simulink model "simulation_Nonlinear_ship_moving_target_ALL"  (R2024b)
settings: Solver=VariableStepAuto  StartTime=0.0  StopTime=30  RelTol=1e-3
libraries: simulink x3
settings Model: Creator=Omer Mizrachi  LastModifiedBy=alonorlicky

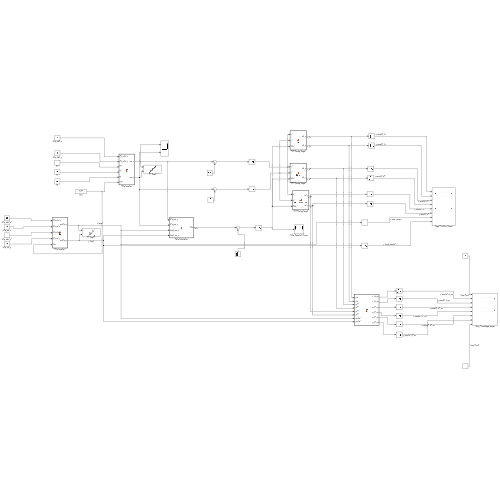
[thumbnail: Simulink's stored preview of the top-level diagram]
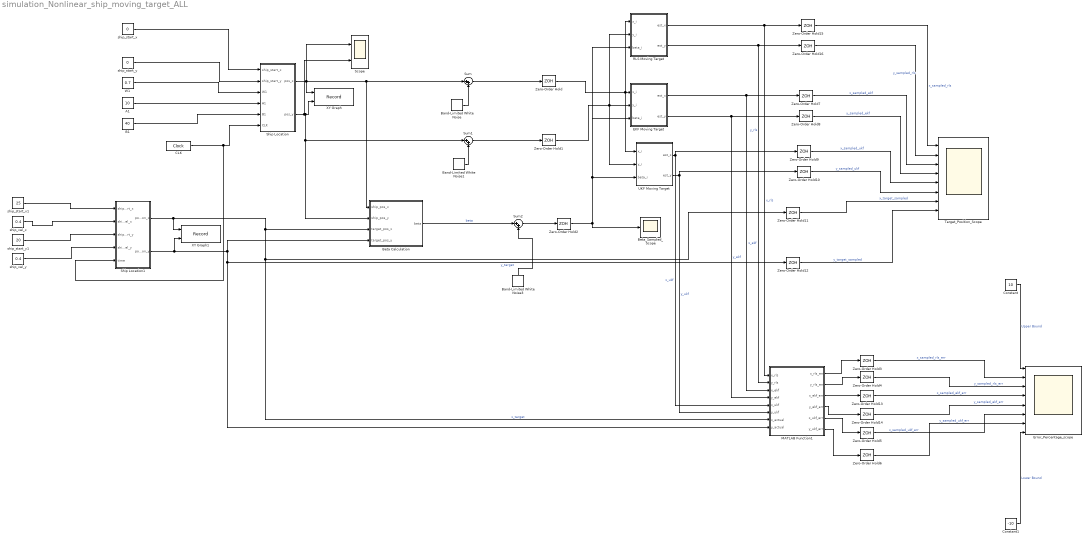
== system simulation_Nonlinear_ship_moving_target_ALL ==
  A1 : Constant  Value=10
  B1 : Constant  Value=40
  Band-Limited White Noise : simulink/Sources/Band-Limited White Noise  Cov=[1.2]  Ts=0.01  seed=[23341]
  Band-Limited White Noise1 : simulink/Sources/Band-Limited White Noise  Cov=[1.2]  Ts=0.01  seed=[233471]
  Band-Limited White Noise3 : simulink/Sources/Band-Limited White Noise  Cov=[ 0.0001]  Ts=0.01  seed=[21113341]
  Beta Calculation : MATLAB Function  TreatAsAtomicUnit=on
  Beta_Sampled_Scope : Scope
  CLK : DigitalClock  SampleTime=0.01
  Constant : Constant  Value=10
  Constant1 : Constant  Value=-10
  EKF Moving Target : MATLAB Function  TreatAsAtomicUnit=on
  Error_Percentage_scope : Scope  NumInputPorts=8
  MATLAB Function1 : MATLAB Function  TreatAsAtomicUnit=on
  RLS Moving Target : MATLAB Function  TreatAsAtomicUnit=on
  Scope : Scope  NumInputPorts=2
  Ship Location : MATLAB Function  TreatAsAtomicUnit=on
  Ship Location1 : MATLAB Function  TreatAsAtomicUnit=on
  Sum : Sum  Inputs=|++
  Sum1 : Sum  Inputs=|++
  Sum2 : Sum  Inputs=|++
  Target_Position_Scope : Scope  NumInputPorts=8
  UKF Moving Target : MATLAB Function  TreatAsAtomicUnit=on
  W1 : Constant  Value=0.7
  XY Graph : Record  FileSettingsInternal="{\"entries\":[{\"content\":{\"excelSettings\":{\"content\":{},\"type\":\"Streamout.ExcelSettings\"}},\"type\":\"Streamout.FileSettingStorage\",\"uuid\":\"\"}],\"packageUris\":[\"http:\\/\\/schema.mathworks.com\\/mf0\\/streamout_blocks\\/R2020a\"],\"version\":\"1.0\"}"  Layout=[1 1]  SignalsInternal="{\"entries\":[{\"content\":{\"signals\":[{\"content\":{\"blockPath\":[],\"dimensions\":[1],\"domain\":\"\",\"lineColor\":\"#0072bd\",\"lineWidth\":2,\"plots\":[ 1 ],\"port\":1,\"sid\":[\"\"],\"signalID\":1,\"signalName\":\"Ship Location:1\"},\"type\":\"RecordBlkView.Signal\",\"uuid\":\"\"},{\"content\":{\"blockPath\":[],\"dimensions\":[1],\"domain\":\"\",\"lineColor\":\"#d95319\",\"lineWidth\":2,\"plots\":[ 1 ],\"port\":2,\"sid\":[\"\"],\"signalID\":2,\"signalName\":\"Ship Location:2\"},\"type\":\"RecordBlkView.Signal\",\"uuid\":\"\"}]},\"type\":\"RecordBlkView.InputSignals\",\"uuid\":\"\"}],\"packageUris\":[\"http:\\/\\/schema.mathworks.com\\/mf0\\/streamout_blocks\\/R2020a\"],\"version\":\"1.0\"}"  VisualizationBindings="{\"xyplotplugin\":{\"info\":[{\"series\":[{\"bindingParametersList\":[{\"parameter\":\"X-Axis\",\"signalID\":1,\"signalName\":\"Ship Location:1\"},{\"parameter\":\"Y-Axis\",\"signalID\":2,\"signalName\":\"Ship Location:2\"}],\"seriesID\":0}],\"subplotID\":1}]}}"  CompatibilityTag=XY
  XY Graph1 : Record  FileSettingsInternal="{\"entries\":[{\"content\":{\"excelSettings\":{\"content\":{},\"type\":\"Streamout.ExcelSettings\"}},\"type\":\"Streamout.FileSettingStorage\",\"uuid\":\"\"}],\"packageUris\":[\"http:\\/\\/schema.mathworks.com\\/mf0\\/streamout_blocks\\/R2020a\"],\"version\":\"1.0\"}"  Layout=[1 1]  SignalsInternal="{\"entries\":[{\"content\":{\"signals\":[{\"content\":{\"blockPath\":[],\"dimensions\":[1],\"domain\":\"\",\"lineColor\":\"#0072bd\",\"lineWidth\":2,\"plots\":[ 1 ],\"port\":1,\"sid\":[\"\"],\"signalID\":1,\"signalName\":\"x_target\"},\"type\":\"RecordBlkView.Signal\",\"uuid\":\"\"},{\"content\":{\"blockPath\":[],\"dimensions\":[1],\"domain\":\"\",\"lineColor\":\"#d95319\",\"lineWidth\":2,\"plots\":[ 1 ],\"port\":2,\"sid\":[\"\"],\"signalID\":2,\"signalName\":\"y_target\"},\"type\":\"RecordBlkView.Signal\",\"uuid\":\"\"}]},\"type\":\"RecordBlkView.InputSignals\",\"uuid\":\"\"}],\"packageUris\":[\"http:\\/\\/schema.mathworks.com\\/mf0\\/streamout_blocks\\/R2020a\"],\"version\":\"1.0\"}"  VisualizationBindings="{\"xyplotplugin\":{\"info\":[{\"series\":[{\"bindingParametersList\":[{\"parameter\":\"X-Axis\",\"signalID\":1,\"signalName\":\"x_target\"},{\"parameter\":\"Y-Axis\",\"signalID\":2,\"signalName\":\"y_target\"}],\"seriesID\":0}],\"subplotID\":1}]}}"  CompatibilityTag=XY
  Zero-Order Hold{,1..16} (17 alike) : ZeroOrderHold  SampleTime=0.01
  ship_start_x : Constant  Value=0
  ship_start_x1 : Constant  Value=25
  ship_start_y : Constant  Value=0
  ship_start_y1 : Constant  Value=20
  ship_vel_x : Constant  Value=0.4
  ship_vel_y : Constant  Value=0.4
  wires:
  Ship Location/2(pos_y) -> Scope/2, Sum1/1, Beta Calculation/2(ship_pos_y), XY Graph/2
  Zero-Order Hold14/1 -> Error_Percentage_scope/5  "y_sampled_ekf_err"
  Zero-Order Hold/1 -> RLS Moving Target/1(x_i), UKF Moving Target/1(x_i), EKF Moving Target/1(x_i)
  Band-Limited White Noise1/1 -> Sum1/2
  EKF Moving Target/2(est_y) -> MATLAB Function1/4(y_ekf), Zero-Order Hold8/1  "y_ekf"
  Zero-Order Hold8/1 -> Target_Position_Scope/4  "y_sampled_ekf"
  Ship Location1/2(position_y) -> XY Graph1/2, MATLAB Function1/8(y_actual), Zero-Order Hold12/1, Beta Calculation/4(target_pos_y)  "y_target"
  Sum2/1 -> Zero-Order Hold2/1
  Zero-Order Hold1/1 -> RLS Moving Target/2(y_i), UKF Moving Target/2(y_i), EKF Moving Target/2(y_i)
  Band-Limited White Noise3/1 -> Sum2/2
  Zero-Order Hold11/1 -> Target_Position_Scope/7  "x_target_sampled"
  MATLAB Function1/3(x_ekf_err) -> Zero-Order Hold13/1
  Ship Location/1(pos_x) -> XY Graph/1, Scope/1, Sum/1, Beta Calculation/1(ship_pos_x)
  Sum1/1 -> Zero-Order Hold1/1
  Zero-Order Hold2/1 -> EKF Moving Target/3(beta_i), RLS Moving Target/3(beta_i), UKF Moving Target/3(beta_i), Beta_Sampled_Scope/1
  Sum/1 -> Zero-Order Hold/1
  Zero-Order Hold13/1 -> Error_Percentage_scope/4  "x_sampled_ekf_err"
  Ship Location1/1(position_x) -> XY Graph1/1, Zero-Order Hold11/1, MATLAB Function1/7(x_actual), Beta Calculation/3(target_pos_x)  "x_target"
  Beta Calculation/1(beta) -> Sum2/1  "beta"
  Zero-Order Hold7/1 -> Target_Position_Scope/3  "x_sampled_ekf"
  Zero-Order Hold12/1 -> Target_Position_Scope/8  "y_target_sampled"
  EKF Moving Target/1(est_x) -> MATLAB Function1/3(x_ekf), Zero-Order Hold7/1  "x_ekf"
  MATLAB Function1/4(y_ekf_err) -> Zero-Order Hold14/1
  Band-Limited White Noise/1 -> Sum/2
  Constant1/1 -> Error_Percentage_scope/8  "Lower Bound"
  Constant/1 -> Error_Percentage_scope/1  "Upper Bound"
  UKF Moving Target/2(est_y) -> MATLAB Function1/6(y_ukf), Zero-Order Hold10/1  "y_ukf"
  UKF Moving Target/1(est_x) -> MATLAB Function1/5(x_ukf), Zero-Order Hold9/1  "x_ukf"
  RLS Moving Target/2(est_y) -> MATLAB Function1/2(y_rls), Zero-Order Hold16/1  "y_rls"
  RLS Moving Target/1(est_x) -> Zero-Order Hold15/1, MATLAB Function1/1(x_rls)  "x_rls"
  Zero-Order Hold4/1 -> Error_Percentage_scope/3  "y_sampled_rls_err"
  MATLAB Function1/2(y_rls_err) -> Zero-Order Hold4/1
  MATLAB Function1/1(x_rls_err) -> Zero-Order Hold3/1
  Zero-Order Hold3/1 -> Error_Percentage_scope/2  "x_sampled_rls_err"
  Zero-Order Hold6/1 -> Error_Percentage_scope/7  "y_sampled_ukf_err"
  MATLAB Function1/6(y_ukf_err) -> Zero-Order Hold6/1
  MATLAB Function1/5(x_ukf_err) -> Zero-Order Hold5/1
  Zero-Order Hold5/1 -> Error_Percentage_scope/6  "x_sampled_ukf_err"
  Zero-Order Hold15/1 -> Target_Position_Scope/1  "x_sampled_rls"
  Zero-Order Hold16/1 -> Target_Position_Scope/2  "y_sampled_rls"
  Zero-Order Hold9/1 -> Target_Position_Scope/5  "x_sampled_ukf"
  Zero-Order Hold10/1 -> Target_Position_Scope/6  "y_sampled_ukf"
  B1/1 -> Ship Location/5(B1)
  ship_start_x/1 -> Ship Location/1(ship_start_x)
  W1/1 -> Ship Location/3(W1)
  ship_start_y/1 -> Ship Location/2(ship_start_y)
  A1/1 -> Ship Location/4(A1)
  CLK/1 -> Ship Location1/5(time), Ship Location/6(CLK)
  ship_start_x1/1 -> Ship Location1/1(ship_start_x)
  ship_vel_y/1 -> Ship Location1/4(ship_vel_y)
  ship_vel_x/1 -> Ship Location1/2(ship_vel_x)
  ship_start_y1/1 -> Ship Location1/3(ship_start_y)

== matlab function simulation_Nonlinear_ship_moving_target_ALL/EKF Moving Target ==
  data: x_i input; est_x output; y_i input; beta_i input; est_y output
function [est_x, est_y] = ekf_fcn(x_i, y_i, beta_i)

persistent X_i P Q R


if isempty(P)
    P = 10*eye(8); % Covariance matrix initialization (8x8)
    Q = 0.1*diag([0.001, 0.001, 0.01, 0.001, 0.01, 0.001, 0.01, 0.001]); % Process noise covariance initialization (8x8)
    R = diag([1, 1, 300]); % Measurement noise covariance initialization (3x3)
end
 
if isempty(X_i)
    X_i = zeros(8, 1); % State vector initialization (8x1)
end

dt = 0.01; % Sample time variable
F = [1 dt 0 0 0 0 0 0 ;
     0 1 0 0 0 0 0 0 ; 
     0 0 1 dt 0 0 0 0 ; 
     0 0 0 1 0 0 0 0 ; 
     0 0 0 0 1 dt 0 0 ; 
     0 0 0 0 0 1 0 0 ; 
     0 0 0 0 0 0 1 dt ; 
     0 0 0 0 0 0 0 1]; % Process Jacobian (8x8)
H = [0 0 0 0 1 0 0 0 ; 
    0 0 0 0 0 0 1 0 ; 
    sin(beta_i) 0 -cos(beta_i) 0 -sin(beta_i) 0 cos(beta_i) 0]; % Measurement Jacobian (3x8)

% Prediction Step
X_i = F*X_i; % Process Model
measurement = [x_i ; y_i ; 0]; % Measurements
predicted_measurement = H*X_i; % Measurement Model
P = F*P*F' + Q; % Covariance matrix

% Update Step
innovation = measurement - predicted_measurement; % Measurement residual
K = P*H'/(H*P*H' + R); % Kalman gain
X_i = X_i + K*innovation; % State vector update
P = (eye(8) - K*H)*P; % Covariance matrix update

% Output estimated position
est_x = X_i(1); % x_t estimation
est_y = X_i(3); % y_t estimation


end

== matlab function simulation_Nonlinear_ship_moving_target_ALL/Beta Calculation ==
  data: ship_pos_x input; beta output; ship_pos_y input; target_pos_x input; target_pos_y input
function beta = fcn(ship_pos_x,ship_pos_y,target_pos_x,target_pos_y)

differ_target_ship_x = target_pos_x - ship_pos_x;
differ_target_ship_y = target_pos_y - ship_pos_y;

beta = atan2(differ_target_ship_y,differ_target_ship_x);

== matlab function simulation_Nonlinear_ship_moving_target_ALL/Ship Location1 ==
  data: ship_start_x input; ship_vel_x input; ship_start_y input; position_x output; ship_vel_y input; time input; position_y output
function [position_x,position_y] = fcn(ship_start_x,ship_vel_x,ship_start_y,ship_vel_y,time)

position_x = ship_start_x + ship_vel_x*time;
position_y = ship_start_y + ship_vel_y*time;

== matlab function simulation_Nonlinear_ship_moving_target_ALL/RLS Moving Target ==
  data: x_i input; est_x output; y_i input; beta_i input; est_y output
function [est_x, est_y] = fcn(x_i, y_i, beta_i)
% fcn - Recursive Least Squares estimator for a 2D moving target using adaptive forgetting factor


    % Persistent variables
    persistent covariance_matrix state_estimate lambda lambda_o

    % Initialization
    if isempty(covariance_matrix)
        covariance_matrix = eye(2);   % Initial covariance matrix
        lambda_o = 0.9;               % forgetting factor
        lambda = 0.6;                 % Initial forgetting factor
    end

    if isempty(state_estimate)
        state_estimate = zeros(2, 1); % Initial position estimate [0; 0]
    end

    % direction vector
    direction_vector = [-sin(beta_i); cos(beta_i)];

    % Project measurement to direction vector
    z_i = y_i * cos(beta_i) - x_i * sin(beta_i);

    % Compute innovation (measurement residual)
    innovation = z_i - direction_vector' * state_estimate;

    % Update state estimate
    gain_denominator = lambda + direction_vector' * covariance_matrix * direction_vector;
    gain_numerator   = covariance_matrix * direction_vector;
    state_estimate   = state_estimate + (gain_numerator / gain_denominator) * innovation;

    % Update covariance matrix
    gain_vector       = covariance_matrix * direction_vector / (lambda + direction_vector' * covariance_matrix * direction_vector);
                        
    covariance_matrix = (1 / lambda) * (covariance_matrix - gain_vector * direction_vector' * covariance_matrix);
                        
    % Adapt forgetting factor
    lambda = lambda_o * lambda + (1 - lambda_o);

    % Output estimated position
    est_x = state_estimate(1);
    est_y = state_estimate(2);
end

== matlab function simulation_Nonlinear_ship_moving_target_ALL/MATLAB Function1 ==
  data: x_rls input; y_rls input; x_rls_err output; y_rls_err output; x_ekf input; x_ekf_err output; y_ekf input; x_ukf input; y_ukf input; x_actual input; y_actual input; y_ekf_err output; x_ukf_err output; y_ukf_err output
function [x_rls_err,y_rls_err,x_ekf_err,y_ekf_err,x_ukf_err,y_ukf_err]= fcn(x_rls,y_rls,x_ekf,y_ekf,x_ukf,y_ukf,x_actual,y_actual)

x_rls_err = ((x_rls - x_actual)/x_actual)*100;
y_rls_err = ((y_rls - y_actual)/y_actual)*100;

x_ekf_err = ((x_ekf - x_actual)/x_actual)*100;
y_ekf_err = ((y_ekf - y_actual)/y_actual)*100;

x_ukf_err = ((x_ukf - x_actual)/x_actual)*100;
y_ukf_err = ((y_ukf - y_actual)/y_actual)*100;

== matlab function simulation_Nonlinear_ship_moving_target_ALL/UKF Moving Target ==
  data: x_i input; est_x output; y_i input; beta_i input; est_y output
function [est_x, est_y] = ukf_dynamic_fcn(x_i, y_i, beta_i)

persistent X_i P Q R lambda alpha beta nx


if isempty(P)
    nx = 8;
    P = 10 * eye(nx);
    Q = 0.01 * diag([0.01, 0.01, 1, 0.01, 1, 0.01, 1, 0.01]);
    R = diag([1, 1, 400]);

    alpha = 1e-3;
    beta = 2;
    lambda = alpha^2 * (nx + 1) - nx;
end

if isempty(X_i)
    X_i = zeros(nx, 1);
end

dt = 0.001;

Wm = [lambda / (nx + lambda); repmat(1 / (2 * (nx + lambda)), 2 * nx, 1)];
Wc = Wm;
Wc(1) = Wc(1) + (1 - alpha^2 + beta);

sigma_points = generate_sigma_points(X_i, P, lambda);

predicted_sigma_points = process_model(sigma_points, dt);
[X_pred, P_pred] = compute_mean_and_covariance(predicted_sigma_points, Wm, Wc, Q);

measured_sigma_points = measurement_model(predicted_sigma_points, beta_i);
[y_pred, Pyy] = compute_mean_and_covariance(measured_sigma_points, Wm, Wc, R);

Pxy = compute_cross_covariance(predicted_sigma_points, measured_sigma_points, X_pred, y_pred, Wc);

K = Pxy / Pyy;

meas = [x_i; y_i; 0];
resid = meas - y_pred;
X_i = X_pred + K * resid;
P = P_pred - K * Pyy * K';

est_x = X_i(1);
est_y = X_i(3);



end

%% Helper Functions

function sigma_points = generate_sigma_points(mean, covariance, lambda)
    nx = length(mean);
    S = chol((nx + lambda) * covariance, 'lower');
    sigma_points = [mean, bsxfun(@plus, mean, S), bsxfun(@minus, mean, S)];
end

function predicted_sigma_points = process_model(sigma_points, dt)
    F = [1 dt 0 0 0 0 0 0; 
         0 1 0 0 0 0 0 0; 
         0 0 1 dt 0 0 0 0; 
         0 0 0 1 0 0 0 0; 
         0 0 0 0 1 dt 0 0; 
         0 0 0 0 0 1 0 0; 
         0 0 0 0 0 0 1 dt; 
         0 0 0 0 0 0 0 1];
    predicted_sigma_points = F * sigma_points;
end

function measured_sigma_points = measurement_model(sigma_points, beta_i)
    H = [0 0 0 0 1 0 0 0;
         0 0 0 0 0 0 1 0;
         sin(beta_i) 0 -cos(beta_i) 0 -sin(beta_i) 0 cos(beta_i) 0];
    measured_sigma_points = H * sigma_points;
end

function [mean_out, covariance] = compute_mean_and_covariance(sigma_points, Wm, Wc, noise_cov)
    mean_out = sigma_points * Wm;
    diff = bsxfun(@minus, sigma_points, mean_out);
    covariance = diff * diag(Wc) * diff' + noise_cov;
end

function Pxy = compute_cross_covariance(predicted_sigma_points, measured_sigma_points, X_pred, y_pred, Wc)
    diff_x = bsxfun(@minus, predicted_sigma_points, X_pred);
    diff_y = bsxfun(@minus, measured_sigma_points, y_pred);
    Pxy = diff_x * diag(Wc) * diff_y';
end

== matlab function simulation_Nonlinear_ship_moving_target_ALL/Ship Location ==
  data: ship_start_x input; pos_x output; ship_start_y input; W1 input; A1 input; B1 input; CLK input; pos_y output
function [pos_x,pos_y] = fcn(ship_start_x,ship_start_y,W1,A1,B1,CLK)


pos_x = A1*cos(W1*CLK) + ship_start_x;
pos_y = B1*sin(W1*CLK) + ship_start_y;
